simulink model "test3"  (R2020b)
settings: Solver=FixedStepAuto  StartTime=0.0  StopTime=10.0  RelTol=1e-3
model workspace (MAT data in the model file):
  HDLVAXIMasterConfig = hdlverifier.internal.AXIMaster.ConfigParams
settings Model: Creator=horse  LastModifiedBy=horse
settings OptimizationCC: BlockReduction=off  ConditionallyExecuteInputs=off  DefaultParameterBehavior=Inlined  OptimizeBlockIOStorage=off
settings HardwareCC: TargetBitPerPointer=64  TargetBitPerSizeT=64  TargetBitPerPtrDiffT=64  TargetLongLongMode=on  TargetIntDivRoundTo=Zero  TargetEndianess=LittleEndian  TargetWordSize=64  TargetHWDeviceType=Generic->Custom  ProdEqTarget=off
settings RTWCC: Description=SystemVerilog DPI Component Generator  SystemTargetFile=systemverilog_dpi_grt.tlc  TemplateMakefile=systemverilog_dpi_grt_default_tmf
settings CodeAppCC: MaxIdLength=256
settings DPIGRTTargetCC: TargetFcnLib=ansi_tfl_table_tmw.mat  GenFloatMathFcnCalls=NOT IN USE  TargetLangStandard=C89/C90 (ANSI)  CodeReplacementLibrary=None  UtilityFuncGeneration=Auto  MultiwordTypeDef=System defined  MultiwordLength=2048  DynamicStringBufferSize=256  GenerateFullHeader=on  InferredTypesCompatibility=off  GenerateSampleERTMain=off  GenerateTestInterfaces=off  ModelReferenceCompliant=on  ParMdlRefBuildCompliant=on  CompOptLevelCompliant=off  ConcurrentExecutionCompliant=off  IncludeMdlTerminateFcn=on  CombineOutputUpdateFcns=off  CombineSignalStateStructs=on  GroupInternalDataByFunction=off  SuppressErrorStatus=off  IncludeFileDelimiter=Auto  ERTCustomFileBanners=off  SupportAbsoluteTime=on  LogVarNameModifier=rt_  MatFileLogging=off  CodeInterfacePackaging=Reusable function  PurelyIntegerCode=off  SupportNonFinite=on  SupportComplex=on  SupportContinuousTime=on  SupportNonInlinedSFcns=on  RemoveDisableFunc=off  RemoveResetFunc=off  SupportVariableSizeSignals=off  ParenthesesLevel=Nominal  CastingMode=Nominal  MATLABClassNameForMDSCustomization=Simulink.SoftwareTarget.TargetSpecificTriggerConfigurationBase  ModelStepFunctionPrototypeControlCompliant=off  CPPClassGenCompliant=off  AutosarCompliant=off  MDXCompliant=off  GRTInterface=off  GenerateAllocFcn=on  UseToolchainInfoCompliant=on  GenerateSharedConstants=on  CoderGroups=[]  AccessMethods=[]  LookupTableObjectStructAxisOrder=1,2,3,4,...  LUTObjectStructOrderExplicitValues=Size,Breakpoints,Table  LUTObjectStructOrderEvenSpacing=Size,Breakpoints,Table  ArrayLayout=Column-major  UnsupportedSFcnMsg=error  ERTHeaderFileRootName=$R$E  ERTSourceFileRootName=$R$E  ERTDataFileRootName=$R_data  RTWCAPISignals=on  RTWCAPIParams=off  RTWCAPIStates=off  RTWCAPIRootIO=off  ExtMode=off  ExtModeTransport=0  ExtModeStaticAlloc=off  ExtModeStaticAllocSize=1000000  ExtModeTesting=off  ExtModeMexFile=ext_comm  GenerateASAP2=off  MultiInstanceErrorCode=Error  DPICustomizeSystemVerilogCode=off  DPISystemVerilogTemplate=svdpi_event.vgt  DPIReportRunTimeError=off  DPIRunTimeErrorSeverity=Fatal  DPIGenerateTestBench=off  DPITestBenchSimulator=Mentor Graphics Questasim  DPITestPointAccessFcnInterface=None  DPIFixedPointDataType=CompatibleCType  DPIPortConnection=Port list  DPICompositeDataType=Flattened

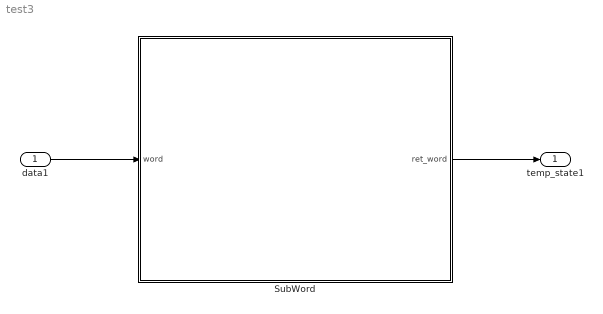
== system test3 ==
  data1 : Inport  OutDataTypeStr=uint32
  SubWord : MATLAB Function  TreatAsAtomicUnit=on
  temp_state1 : Outport  OutDataTypeStr=uint32  VectorParamsAs1DForOutWhenUnconnected=off
  wires:
  data1/1 -> SubWord/1(word)
  SubWord/1(ret_word) -> temp_state1/1

== matlab function test3/SubWord ==
  data: ret_word output; word input
function ret_word  = SubWord(word)

    % did not mess with indexing

	%sub byte
	%uint8_t words[4] = { 0 };
%     words = uint8(zeros(1,4));
% 	words = BreakWordDown(words, word);
    words = uint32([0 0 0 0]);
    
    words(4) = getSBoxValue(uint8(bitsrl(bitand(word, 0xFF000000), 24)));
    
    words(3) = getSBoxValue(uint8(bitsrl(bitsll(bitand(word, 0x00FF0000), 8), 24)));
    
    words(2) = getSBoxValue(uint8(bitsrl(bitsll(bitand(word, 0x0000FF00), 16), 24)));
    
    words(1) = getSBoxValue(uint8(bitsrl(bitsll(bitand(word, 0x000000FF), 24), 24)));
        
    ret_word = uint32(0);
    ret_word = ret_word + words(4);
    ret_word = bitsll(ret_word, 8);
	ret_word = ret_word + words(3);
	ret_word = bitsll(ret_word, 8);
	ret_word = ret_word + words(2);
	ret_word = bitsll(ret_word, 8);
	ret_word = ret_word + words(1);
end
